simulink model "sfcndemo_stspace"  (Simulink 7.6)
settings: Solver=ode3  StartTime=0.0  StopTime=10.0  RelTol=1e-3
Description:
  | Continuous-Time State-Space C-MEX S-function
settings Model: Creator=The MathWorks Inc.  ExtModeTrigMode=oneshot  ExtModeArmWhenConnect=off  ExtModeAutoUpdateStatusClock=off
settings DataIOCC: LimitDataPoints=off
settings OptimizationCC: BlockReduction=off  BooleanDataType=off  InitFltsAndDblsToZero=on
settings DebuggingCC: SaveWithParameterizedLinksMsg=none  SignalResolutionControl=TryResolveAllWithWarning  SolverPrmCheckMsg=none  MultiTaskDSMMsg=warning  MultiTaskCondExecSysMsg=none
settings HardwareCC: TargetUnknown=on
settings RTWCC: IncludeERTFirstTime=on
settings CodeAppCC: CustomSymbolStrFcn=$F$N$M
settings GRTTargetCC: TargetFcnLib=ansi_tfl_tmw.mat

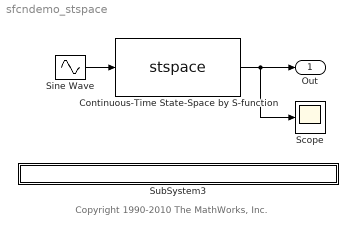
== system sfcndemo_stspace ==
  note: Copyright 1990-2010 The MathWorks, Inc.
  Continuous-Time State-Space by S-function : S-Function  FunctionName=stspace  Parameters=a,b,c,d,x0  EnableBusSupport=off  mask(S-function: stspace){a=[-0.09 -0.01; 1 0], b=[1 -7; 0 -2], c=[0 2; 1 -5], d=[-3 0; 1 0], x0=[]}
      mask prompts: x0 "Initial condition:"
      mask help: This is a S-function block which is the state-space system with dynamic inputs, outputs and states.
      mask Display: disp('dx/dt = A*X + B*U\n Y      = C*X + D*U ');
  Scope : Scope
      settings: TimeRange=10  YMin=-200  YMax=500
  Sine Wave : Sin  Amplitude=[1 2]  SampleTime=0
  SubSystem3 : Subsystem  mask{filename=stspace.c}
      mask init:
      | x=sfundemo_maskdisp;
      settings: AttributesFormatString=\n  OpenFcn=sfundemo_openfcn
      mask Display: disp(x);
  Out : Outport  InitialOutput=0
  wires:
  Sine Wave/1 -> Continuous-Time State-Space by S-function/1
  Continuous-Time State-Space by S-function/1 -> Out/1, Scope/1

== system sfcndemo_stspace/SubSystem3 ==
